simulink model "Sim_Path_Forces2"  (R2016a)
settings: Solver=VariableStepAuto  StartTime=0.0  StopTime=60  RelTol=1e-3
values from neighbouring files (symbols this model uses):
  ad = 0.1031    [Initial_conitions.m]    (also in alpha_equation.m)
  al = 0.8671    [Initial_conitions.m]    (also in alpha_equation.m)
  bd = 4.2706    [Initial_conitions.m]    (also in alpha_equation.m)
  bl = 7.1112    [Initial_conitions.m]    (also in alpha_equation.m)
  dynamic0 = [Vtot gamma chi hn phin thetan mf psiV psigamma     psichi psih psiphi psitheta psim]'    [Initial_conitions.m]
libraries: aerolibconvert2 x5
settings Model: Creator=Bakry  LastModifiedBy=Bakry

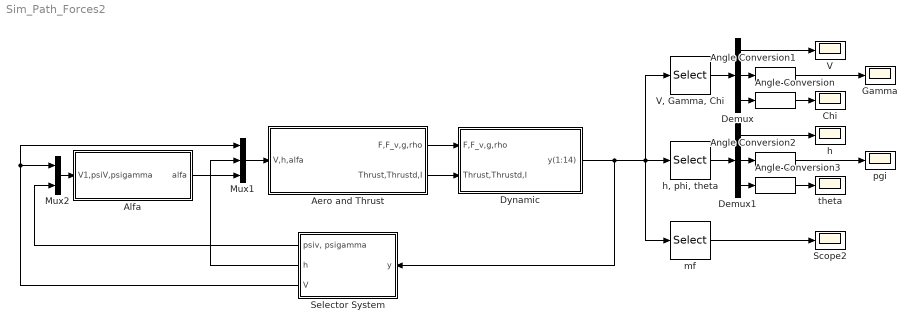
== system Sim_Path_Forces2 ==
  Aero and Thrust : Subsystem
  Alfa : Subsystem
  Angle Conversion{,1..3} (4 alike) : aerolibconvert2/Angle Conversion  IU=rad  OU=deg
  Chi : Scope
  Demux : Demux  Outputs=3
  Demux1 : Demux  Outputs=3
  Dynamic : Subsystem
  Gamma : Scope
  Mux1 : Mux  Inputs=3
  Mux2 : Mux  Inputs=2
  Scope2 : Scope
  Selector System : Subsystem
  V : Scope
  "V, Gamma, Chi" : Selector  InputPortWidth=14  IndexOptions=Index vector (dialog)  Indices=[1 2 3]  OutputSizes=1
  h : Scope
  "h, phi, theta" : Selector  InputPortWidth=14  IndexOptions=Index vector (dialog)  Indices=[4 5 6]  OutputSizes=1
  mf : Selector  InputPortWidth=14  IndexOptions=Index vector (dialog)  Indices=[7]  OutputSizes=1
  pgi : Scope
  theta : Scope
  wires:
  Aero and Thrust/2(Thrust,Thrustd,I) -> Dynamic/2(Thrust,Thrustd,I)
  Aero and Thrust/1(F,F_v,g,rho) -> Dynamic/1(F,F_v,g,rho)
  Mux1/1 -> Aero and Thrust/1(V,h,alfa)
  Alfa/1(alfa) -> Mux1/3
  "V, Gamma, Chi"/1 -> Demux/1
  Demux/2 -> Angle Conversion1/1
  Demux/3 -> Angle Conversion/1
  Demux/1 -> V/1
  Dynamic/1(y(1:14)) -> "V, Gamma, Chi"/1, mf/1, "h, phi, theta"/1, Selector System/1(y)
  "h, phi, theta"/1 -> Demux1/1
  Demux1/3 -> Angle Conversion3/1
  Demux1/1 -> h/1
  mf/1 -> Scope2/1
  Mux2/1 -> Alfa/1(V1,psiV,psigamma)
  Selector System/1("psiv, psigamma") -> Mux2/2
  Selector System/2(h) -> Mux1/2
  Selector System/3(V) -> Mux2/1, Mux1/1
  Angle Conversion/1 -> Chi/1
  Angle Conversion1/1 -> Gamma/1
  Demux1/2 -> Angle Conversion2/1
  Angle Conversion2/1 -> pgi/1
  Angle Conversion3/1 -> theta/1

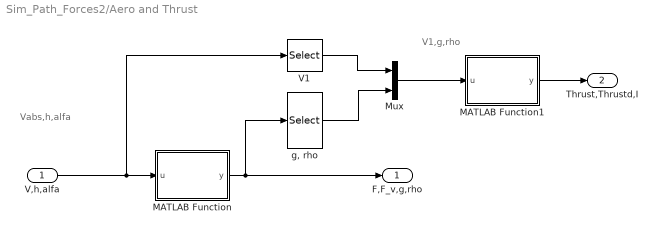
== system Sim_Path_Forces2/Aero and Thrust ==
  note: Vabs,h,alfa
  note: V1,g,rho
  V,h,alfa : Inport
  MATLAB Function : MATLAB Function  TreatAsAtomicUnit=on
  MATLAB Function1 : MATLAB Function  TreatAsAtomicUnit=on
  Mux : Mux  Inputs=2
  V1 : Selector  InputPortWidth=3  IndexOptions=Index vector (dialog)  Indices=[1]  OutputSizes=1
  "g, rho" : Selector  InputPortWidth=8  IndexOptions=Index vector (dialog)  Indices=[7 8]  OutputSizes=1
  F,F_v,g,rho : Outport
  Thrust,Thrustd,I : Outport  Port=2
  wires:
  MATLAB Function/1(y) -> "g, rho"/1, F,F_v,g,rho/1
  Mux/1 -> MATLAB Function1/1(u)
  V1/1 -> Mux/1
  "g, rho"/1 -> Mux/2
  MATLAB Function1/1(y) -> Thrust,Thrustd,I/1
  V,h,alfa/1 -> MATLAB Function/1(u), V1/1

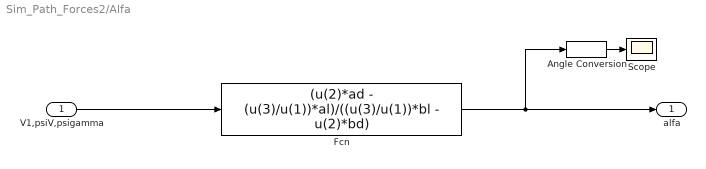
== system Sim_Path_Forces2/Alfa ==
  V1,psiV,psigamma : Inport
  Angle Conversion : aerolibconvert2/Angle Conversion  IU=rad  OU=deg
  Fcn : Fcn  Expr=(u(2)*ad - (u(3)/u(1))*al)/((u(3)/u(1))*bl - u(2)*bd)
  Scope : Scope
  alfa : Outport
  wires:
  V1,psiV,psigamma/1 -> Fcn/1
  Fcn/1 -> alfa/1, Angle Conversion/1
  Angle Conversion/1 -> Scope/1

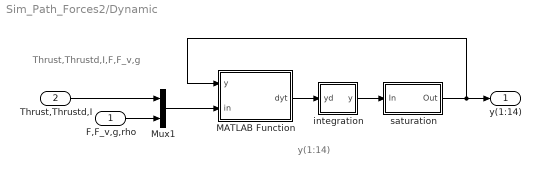
== system Sim_Path_Forces2/Dynamic ==
  note: Thrust,Thrustd,I,F,F_v,g
  note: y(1:14)
  F,F_v,g,rho : Inport
  Thrust,Thrustd,I : Inport  Port=2
  MATLAB Function : MATLAB Function  TreatAsAtomicUnit=on
  Mux1 : Mux  Inputs=2
  integration : Subsystem
  saturation : Subsystem
  y(1:14) : Outport
  wires:
  MATLAB Function/1(dyt) -> integration/1(yd)
  integration/1(y) -> saturation/1(In)
  Thrust,Thrustd,I/1 -> Mux1/1
  Mux1/1 -> MATLAB Function/2(in)
  F,F_v,g,rho/1 -> Mux1/2
  saturation/1(Out) -> MATLAB Function/1(y), y(1:14)/1

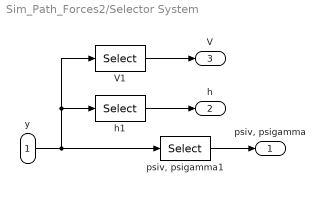
== system Sim_Path_Forces2/Selector System ==
  y : Inport
  V1 : Selector  InputPortWidth=14  IndexOptions=Index vector (dialog)  Indices=[1]  OutputSizes=1
  h1 : Selector  InputPortWidth=14  IndexOptions=Index vector (dialog)  Indices=[4]  OutputSizes=1
  "psiv, psigamma1" : Selector  InputPortWidth=14  IndexOptions=Index vector (dialog)  Indices=[8 9]  OutputSizes=1
  "psiv, psigamma" : Outport
  h : Outport  Port=2
  V : Outport  Port=3
  wires:
  "psiv, psigamma1"/1 -> "psiv, psigamma"/1
  h1/1 -> h/1
  y/1 -> "psiv, psigamma1"/1, V1/1, h1/1
  V1/1 -> V/1

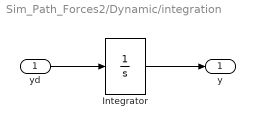
== system Sim_Path_Forces2/Dynamic/integration ==
  yd : Inport
  Integrator : Integrator  InitialCondition=dynamic0
  y : Outport
  wires:
  yd/1 -> Integrator/1
  Integrator/1 -> y/1

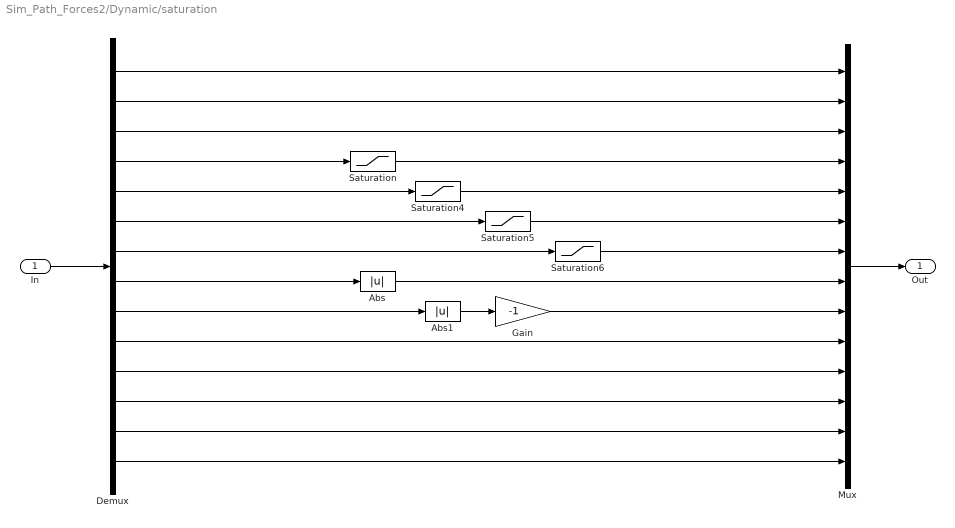
== system Sim_Path_Forces2/Dynamic/saturation ==
  In : Inport
  Abs : Abs
  Abs1 : Abs
  Demux : Demux  Outputs=14
  Gain : Gain  Gain=-1
  Mux : Mux  Inputs=14
  Saturation : Saturate  UpperLimit=30001  LowerLimit=29999
  Saturation4 : Saturate  UpperLimit=1.4  LowerLimit=-1.4
  Saturation5 : Saturate  UpperLimit=3.1415  LowerLimit=-3.1415
  Saturation6 : Saturate  UpperLimit=81646.63  LowerLimit=0
  Out : Outport
  wires:
  In/1 -> Demux/1
  Demux/4 -> Saturation/1
  Saturation/1 -> Mux/4
  Demux/1 -> Mux/1
  Demux/2 -> Mux/2
  Demux/3 -> Mux/3
  Demux/5 -> Saturation4/1
  Saturation4/1 -> Mux/5
  Demux/6 -> Saturation5/1
  Saturation5/1 -> Mux/6
  Demux/7 -> Saturation6/1
  Saturation6/1 -> Mux/7
  Demux/9 -> Abs1/1
  Demux/10 -> Mux/10
  Demux/11 -> Mux/11
  Demux/12 -> Mux/12
  Demux/13 -> Mux/13
  Demux/14 -> Mux/14
  Mux/1 -> Out/1
  Demux/8 -> Abs/1
  Abs/1 -> Mux/8
  Abs1/1 -> Gain/1
  Gain/1 -> Mux/9

== matlab function Sim_Path_Forces2/Aero and Thrust/MATLAB Function1 ==
  data: u input; y output
function y = fcn(u)

Ac     = 27.87;
a      = 305;

V1 = u(1);
g = u(2);
rho = u(3);

Mach = V1/a;
[I,dI1,dI2,p,pd]=Engine_CT(Mach);

CTP  = polyval(p,Mach);
CTPd = polyval(pd,Mach);

Thrust  = 0.029*rho*g*V1*I*Ac*CTP;
Thrustd = 0.029*rho*g*dI1*Ac*CTP*V1 + 0.029*rho*g*I*Ac*CTPd*V1 +... 
          0.029*rho*g*(1/a)*I*Ac*CTP;

y = [Thrust Thrustd I];

== matlab function Sim_Path_Forces2/Aero and Thrust/MATLAB Function ==
  data: u input; y output
function y = fcn(u)
Sref   = 21.672;
rhos   = 1.225;
gs     = 9.80665;
bet    = 0.000140845;
rearth = 6.38E6;


arc = pi/180.;

Vabs = u(1);
h = u(2);
alfa = u(3);

% ********************************************************
% Generation of Aerodynamics of Space Vehicle
% ********************************************************

R = h + rearth;
beta = 0;

rho = rhos*exp(-bet*h);
% H = 10351.8-(0.0368512).*h-(1.02368e-5).*h.^2+(2.63363e-10).*h.^3;
% rho = rhos.*exp(-h./H);
g   = gs*(rearth/R)^2;

norm = rho/2.*Vabs^2*Sref;
norm2 = rho.*Vabs*Sref;

% algr = alfa/arc;
% begr = beta/arc;

% ********************************************************
% X-38 Longitudinal and Lateral Aerodynamics
% ********************************************************

CL = -0.0057 + 0.8671*alfa + 3.5556*alfa^2;
CD = -0.0101 + 0.1031*alfa + 2.1353*alfa^2;
CQ =  0.0000 - 0.1038*beta + 0.0299*beta^2;

D = norm*CD;
Y = norm*CQ;
L = norm*CL;
F = [D Y L];
Dv = norm2*CD;
Yv = norm2*CQ;
Lv = norm2*CL;
F_v = [Dv Yv Lv];

y = [D Y L Dv Yv Lv g rho];

== matlab function Sim_Path_Forces2/Dynamic/MATLAB Function ==
  data: y input; dyt output; in input
function dyt = fcn(y,in)
%*********************************************************************
% Constants
%*********************************************************************
m0      = 136077.7;% Takeoff weight;
omegae = 0.00007292;
rearth = 6.38E6;

%*********************************************************************
% Assigning Variables
%*********************************************************************
V1      = y(1);    gamma1  = y(2);    chi1    = y(3);
h1      = y(4);   phi1    = y(5);   theta1  = y(6);
mf      = y(7);   

psiV    = y(8);    psigamma= y(9);    psichi  = y(10);
psih      = y(11); psiphi= y(12);     psitheta  = y(13);
psim      = y(14); 

Thrust = in(1);   Thrustd = in(2);    I = in(3);
F = in(4:6);      F_v = in (7:9);     g = in(10);
rho = in(10);


% % ********************************************************
% % Estimation of Position
% % ********************************************************
R = h1 + rearth;
h1p     = V1*sin(gamma1);
phi1p   = V1*cos(gamma1)*cos(chi1)/R;
theta1p = V1*cos(gamma1)*sin(chi1)/(R*cos(phi1));

% ***************************************************************
% Mass Consuming Equation 
% ***************************************************************

mfd = - Thrust/(g*I);
m = m0 - mf; 

% ***************************************************************
% Set up of Right Hand Side Eauations
% ***************************************************************

D = F(1); Y = F(2); L = F(3); mu = 0; 
BB = zeros(1,3);
BB(1)=((Thrust-D)/m)-g*sin(gamma1)+omegae^2*R*cos(phi1)^2*...
    (sin(gamma1)-cos(gamma1)*tan(phi1)*sin(chi1));
BB(2)=(1/V1)*((L*cos(mu)-Y*sin(mu))/m - g*cos(gamma1)+(V1^2*...
    cos(gamma1))/R+2*omegae*V1*cos(phi1)*cos(chi1)+omegae^2*R*...
    cos(phi1)^2*(cos(gamma1)+sin(gamma1)*tan(phi1)*sin(chi1)));
BB(3)=(1/V1)*((L*sin(mu)+Y*cos(mu))/(m*cos(gamma1))-(V1^2/R)*cos(gamma1)...
    *cos(chi1)*tan(phi1)+2*omegae*V1*(tan(gamma1)*cos(phi1)*sin(chi1)...
    -sin(phi1))-(omegae^2*R/cos(gamma1))*sin(phi1)*cos(phi1)*cos(chi1));

x1 = [BB(1) BB(2) BB(3)]';

% ***************************************************************
% Complete Set of the 7 Ordinary Differential Equations
% ***************************************************************
dydt = zeros(1,14);
dydt(1) = x1(1);
dydt(2) = x1(2);
dydt(3) = x1(3);

dydt(4) = h1p;
dydt(5) = phi1p;
dydt(6) = theta1p;  
dydt(7) = mfd;

%****************************************************************
% Alpha Costate 7 Differential Equations  
%**************************************************************** 
Dv = F_v(1); Yv = F_v(2); Lv = F_v(3);

psiVd = -psiV*(1/m)*(Thrustd-Dv) - psigamma*((1/(m*V1))*Lv +...
    cos(gamma1)/R + (1/V1^2)*(g*cos(gamma1)-R*omegae^2*cos(phi1)^2*...
    (sin(gamma1)*tan(phi1)*sin(chi1)+cos(gamma1))-L/m))-psichi*...
    (-cos(gamma1)*tan(phi1)*cos(chi1)/R + (omegae^2*R*sin(phi1)*...
    cos(phi1)*cos(chi1))/(cos(gamma1)*V1^2))...
    - psih*sin(gamma1) - psiphi*...
    (cos(gamma1)*cos(chi1)/R) - psitheta*(cos(gamma1)*sin(chi1)/...
    (R*cos(phi1)));

psigammad = -psiV*(-g*cos(gamma1)+R*omegae^2*cos(phi1)^2*(sin(gamma1)*...
    tan(phi1)*sin(chi1)+cos(gamma1))) - psigamma*(R*omegae^2*cos(phi1)...
    ^2*(cos(gamma1)*tan(phi1)*sin(chi1)-sin(gamma1))/V1+sin(gamma1)*...
    (g/V1-V1/R)) - psichi*(-R*omegae^2*sin(phi1)*cos(phi1)*cos(chi1)*...
    sin(gamma1)/(V1*cos(gamma1)^2)+2*omegae*cos(phi1)*sin(chi1)*...
    (tan(gamma1)^2+1)+V1*sin(gamma1)*cos(chi1)*tan(phi1)/R) - psih*...
    (V1*cos(gamma1)) + psiphi*...
    (V1*sin(gamma1)*cos(chi1)/R) + psitheta*(V1*sin(gamma1)*sin(chi1)/...
    (R*cos(phi1)));

psichid = psiV*(R*omegae^2*cos(phi1)^2*cos(gamma1)*tan(phi1)*cos(chi1))-...
    psigamma*(-2*omegae*cos(phi1)*sin(chi1)+R*omegae^2*cos(phi1)^2*...
    sin(gamma1)*tan(phi1)*cos(chi1)/V1) - psichi*(V1*cos(gamma1)*...
    sin(chi1)*tan(phi1)/R+2*omegae*tan(gamma1)*cos(phi1)*cos(chi1)+...
    omegae^2*R*sin(phi1)*cos(phi1)*sin(chi1)/(V1*cos(gamma1))) +...
    psiphi*(V1*cos(gamma1)*...
    sin(chi1)/R) - psitheta*(V1*cos(gamma1)*cos(chi1)/(R*cos(phi1)));

psihd = -psiV*(omegae^2*cos(phi1)^2*(-cos(gamma1)*tan(phi1)*sin(chi1)+...
    sin(gamma1))) - psigamma*(-V1*cos(gamma1)/R^2+omegae^2*cos(phi1)^2*(...
    cos(gamma1)+sin(gamma1)*tan(phi1)*sin(chi1))) - psichi*(V1*cos(...
    gamma1)*cos(chi1)*tan(phi1)/R^2-omegae^2*sin(phi1)*cos(phi1)*...
    cos(chi1)/(V1*cos(gamma1))) + psiphi*(V1*cos(gamma1)*cos(chi1)/R^2)...
    + psitheta*(V1*cos(gamma1)*cos(chi1)/(R^2*cos(phi1)));

psiphid = -psiV*R*omegae^2*(-cos(gamma1)*sin(phi1)^2*sin(chi1)+2*...
    cos(gamma1)*sin(phi1)^2*sin(chi1)-cos(gamma1)*cos(phi1)^2*sin(chi1)-...
    sin(gamma1)*sin(2*phi1)) - psigamma*(-2*omegae*sin(phi1)*cos(chi1)...
    +(R*omegae^2/V1)*(-sin(2*phi1)*cos(gamma1)-sin(2*phi1)*sin(gamma1)*...
    tan(phi1)*sin(chi1)+cos(phi1)^2*sin(gamma1)*sin(chi1)+sin(phi1)^2*...
    sin(gamma1)*sin(chi1))) - psichi*(-V1*cos(gamma1)*cos(chi1)*(tan...
    (phi1)^2+1)/R-2*omegae*(tan(gamma1)*sin(phi1)*sin(chi1)+cos(phi1))...
    +R*omegae^2*cos(chi1)*(sin(phi1)^2-cos(phi1)^2)/(V1*cos(gamma1))) +...
    psitheta*(V1*cos(gamma1)*sin(chi1)*sin(phi1)/(R*cos(phi1)^2));

psithetad = 0;

psimd = - psiV*((-Thrust+D)/m^2) + psigamma*(L/(V1*m^2));

dydt(8) = psiVd;
dydt(9) = psigammad;
dydt(10) = psichid;
dydt(11) = psihd;
dydt(12) = psiphid;
dydt(13) = psithetad;
dydt(14) = psimd;

dyt = double(dydt');

% ***************************************************************
% End of Sub Program RHS
% ***************************************************************
